simulink library "lib_Convection_SphereCrossFlowWhitaker"  (R2015a)
settings: Solver=ode45  StartTime=0.0  StopTime=10.0  RelTol=1e-3
libraries: simulink x6
settings Model: Creator=jlkratz  LastModifiedBy=jlkratz

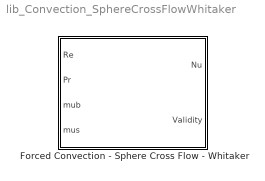
== system lib_Convection_SphereCrossFlowWhitaker ==
  Forced Convection - Sphere Cross Flow - Whitaker : Subsystem  mask(TSAT: Sphere Cross Flow - Whitaker){}
      mask help:
      | This block estimates the average Nusselt number of an external flow over an isothermal sphere using an empirical correlation developed by Whitaker. The Reynolds number (Re) should be calculated based on the diameter of the sphere. Note that all fluid properrties should be evaluated at freestream temperature except for mus which is the vicosity of the fluid evaluated at the surface temperature of the sphere. The correlation is subject to the following restrictions:
      |
      | 3.5 <= Re <= 76000
      | 0.71 <= Pr <= 380
      | 1.0 <= mu/mus <= 3.2
      |
      | Pr is the Prandtl number, and mu is the viscosity. For more information see the block help menu.
      mask Help: web(which('Convection_TSAT_SphereCrossFlowWhitaker.html'),'-helpbrowser')

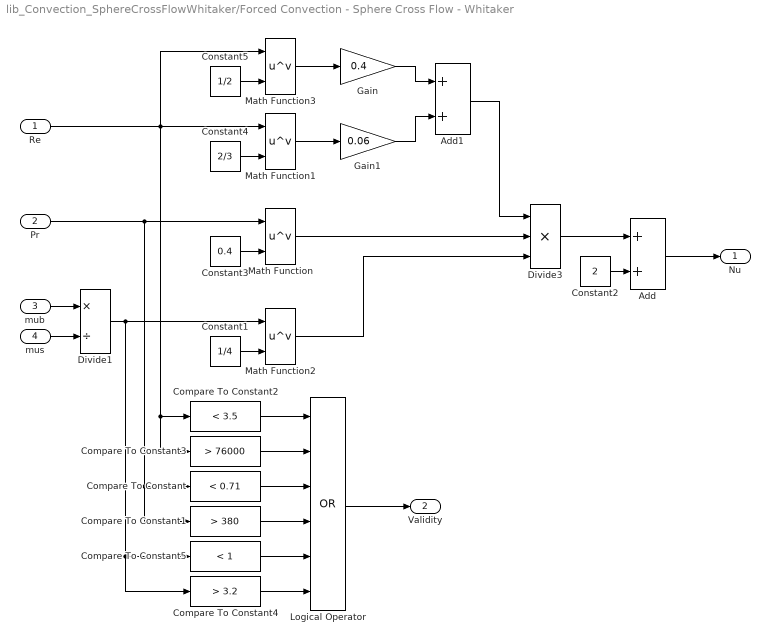
== system lib_Convection_SphereCrossFlowWhitaker/Forced Convection - Sphere Cross Flow - Whitaker ==
  Re : Inport
  Pr : Inport  Port=2
  mub : Inport  Port=3
  mus : Inport  Port=4
  Add : Sum
  Add1 : Sum
  Compare To Constant : simulink/Logic and Bit Operations/Compare To Constant  relop=<  const=0.71  OutDataTypeStr=boolean
  Compare To Constant1 : simulink/Logic and Bit Operations/Compare To Constant  relop=>  const=380  OutDataTypeStr=boolean
  Compare To Constant2 : simulink/Logic and Bit Operations/Compare To Constant  relop=<  const=3.5  OutDataTypeStr=boolean
  Compare To Constant3 : simulink/Logic and Bit Operations/Compare To Constant  relop=>  const=76000  OutDataTypeStr=boolean
  Compare To Constant4 : simulink/Logic and Bit Operations/Compare To Constant  relop=>  const=3.2  OutDataTypeStr=boolean
  Compare To Constant5 : simulink/Logic and Bit Operations/Compare To Constant  relop=<  const=1  OutDataTypeStr=boolean
  Constant1 : Constant  Value=1/4
  Constant2 : Constant  Value=2
  Constant3 : Constant  Value=0.4
  Constant4 : Constant  Value=2/3
  Constant5 : Constant  Value=1/2
  Divide1 : Product  Inputs=*/
  Divide3 : Product  Inputs=***
  Gain : Gain  Gain=0.4
  Gain1 : Gain  Gain=0.06
  Logical Operator : Logic  Operator=OR  Inputs=6  AllPortsSameDT=off  OutDataTypeStr=boolean
  Math Function{,1..3} (4 alike) : Math  Operator=pow  SaturateOnIntegerOverflow=on
  Nu : Outport
  Validity : Outport  Port=2
  wires:
  Add1/1 -> Divide3/1
  Gain1/1 -> Add1/2
  Gain/1 -> Add1/1
  Math Function1/1 -> Gain1/1
  Math Function3/1 -> Gain/1
  Constant5/1 -> Math Function3/2
  Add/1 -> Nu/1
  Divide3/1 -> Add/1
  Constant2/1 -> Add/2
  Constant1/1 -> Math Function2/2
  Compare To Constant5/1 -> Logical Operator/5
  Compare To Constant4/1 -> Logical Operator/6
  Divide1/1 -> Compare To Constant4/1, Compare To Constant5/1, Math Function2/1
  mus/1 -> Divide1/2
  mub/1 -> Divide1/1
  Compare To Constant1/1 -> Logical Operator/4
  Math Function2/1 -> Divide3/3
  Logical Operator/1 -> Validity/1
  Compare To Constant/1 -> Logical Operator/3
  Compare To Constant3/1 -> Logical Operator/2
  Compare To Constant2/1 -> Logical Operator/1
  Math Function/1 -> Divide3/2
  Constant4/1 -> Math Function1/2
  Constant3/1 -> Math Function/2
  Pr/1 -> Compare To Constant/1, Compare To Constant1/1, Math Function/1
  Re/1 -> Math Function1/1, Compare To Constant2/1, Compare To Constant3/1, Math Function3/1
